simulink model "lab1"  (Simulink 7.8)
settings: Solver=ode45  StartTime=0.0  StopTime=100.0  RelTol=1e-3
settings Model: Creator=irina  LastModifiedBy=irina
settings DebuggingCC: SolverPrmCheckMsg=none

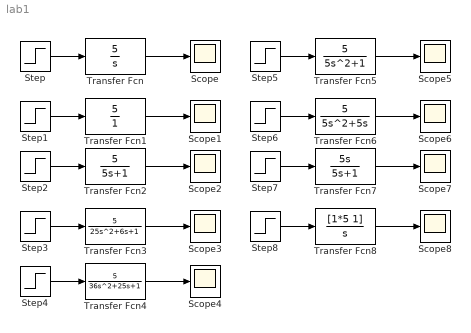
== system lab1 ==
  Scope{,1..8} (9 alike) : Scope
      Scope2 settings: SaveName=ScopeData2
      Scope3 settings: SaveName=ScopeData3
      Scope4 settings: SaveName=ScopeData4
      Scope5 settings: SaveName=ScopeData5
      Scope6 settings: SaveName=ScopeData6
      Scope7 settings: SaveName=ScopeData7
      Scope8 settings: SaveName=ScopeData8
  Step{,1..8} (9 alike) : Step  SampleTime=0
  Transfer Fcn : TransferFcn  Numerator=[5]  Denominator=[1 0]
  Transfer Fcn1 : TransferFcn  Numerator=[5]  Denominator=[1]
  Transfer Fcn2 : TransferFcn  Numerator=[5]  Denominator=[5 1]
  Transfer Fcn3 : TransferFcn  Numerator=[5]  Denominator=[25 6 1]
  Transfer Fcn4 : TransferFcn  Numerator=[5]  Denominator=[36 25 1]
  Transfer Fcn5 : TransferFcn  Numerator=[5]  Denominator=[5 0 1]
  Transfer Fcn6 : TransferFcn  Numerator=[5]  Denominator=[5 5 0]
  Transfer Fcn7 : TransferFcn  Numerator=[5 0]  Denominator=[5 1]
  Transfer Fcn8 : TransferFcn  Numerator=[1*5 1]  Denominator=[1 0]
  wires:
  Step/1 -> Transfer Fcn/1
  Transfer Fcn/1 -> Scope/1
  Step1/1 -> Transfer Fcn1/1
  Transfer Fcn1/1 -> Scope1/1
  Step2/1 -> Transfer Fcn2/1
  Transfer Fcn2/1 -> Scope2/1
  Step3/1 -> Transfer Fcn3/1
  Transfer Fcn3/1 -> Scope3/1
  Step4/1 -> Transfer Fcn4/1
  Transfer Fcn4/1 -> Scope4/1
  Step5/1 -> Transfer Fcn5/1
  Transfer Fcn5/1 -> Scope5/1
  Step6/1 -> Transfer Fcn6/1
  Transfer Fcn6/1 -> Scope6/1
  Step7/1 -> Transfer Fcn7/1
  Transfer Fcn7/1 -> Scope7/1
  Step8/1 -> Transfer Fcn8/1
  Transfer Fcn8/1 -> Scope8/1
